simulink model "ex3_c"  (R2020a)
settings: Solver=VariableStepAuto  StartTime=0.0  StopTime=10.0  RelTol=1e-3
settings Model: Creator=Tomo  LastModifiedBy=Tomo

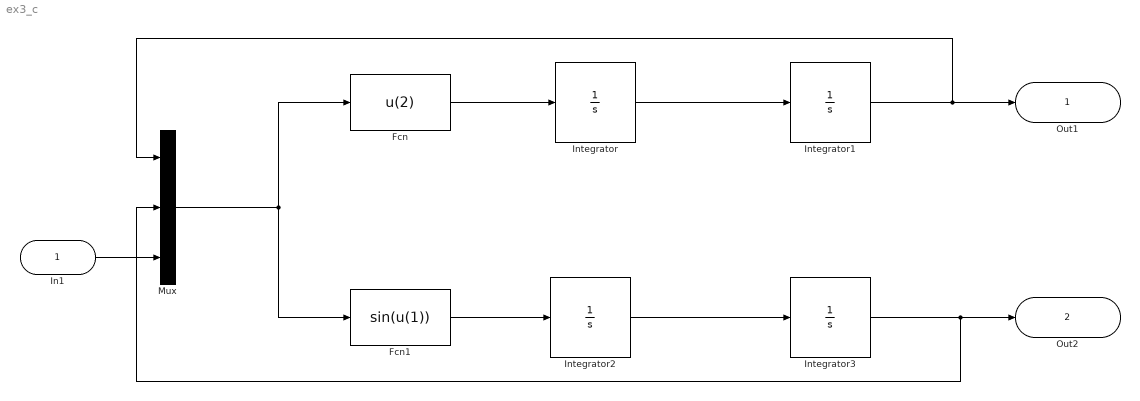
== system ex3_c ==
  In1 : Inport
  Fcn : Fcn  Expr=u(2)
  Fcn1 : Fcn  Expr=sin(u(1))
  Integrator{,1..3} (4 alike) : Integrator
  Mux : Mux  Inputs=3
  Out1 : Outport
  Out2 : Outport  Port=2
  wires:
  Integrator/1 -> Integrator1/1
  Integrator3/1 -> Mux/2, Out2/1
  Integrator2/1 -> Integrator3/1
  Integrator1/1 -> Mux/1, Out1/1
  Mux/1 -> Fcn1/1, Fcn/1
  Fcn/1 -> Integrator/1
  Fcn1/1 -> Integrator2/1
  In1/1 -> Mux/3
